simulink model "sldemo_mdlref_variants_enum"  (Simulink 7.6)
settings: Solver=FixedStepDiscrete  StartTime=0.0  StopTime=10.0  RelTol=1e-3
PreLoadFcn:
  | VE_NONLINEAR_CONTROLLER=Simulink.Variant('E_CTRL==sldemo_mrv_CONTROLLER_TYPE.NONLINEAR')
  | VE_SECOND_ORDER_CONTROLLER=Simulink.Variant('E_CTRL==sldemo_mrv_CONTROLLER_TYPE.SECOND_ORDER')
  | 
  | E_CTRL=sldemo_mrv_CONTROLLER_TYPE.SECOND_ORDER
  | 
  | VE_PROTOTYPE = Simulink.Variant('E_CURRENT_BUILD==sldemo_mrv_BUILD_TYPE.PROTOTYPE')
  | VE_PRODUCTION = Simulink.Variant('E_CURRENT_BUILD==sldemo_mrv_BUILD_TYPE.PRODUCTION')
  | 
  | E_CURRENT_BUILD=sldemo_mrv_BUILD_TYPE.PRODUCTION
settings Model: Creator=The MathWorks Inc.
settings DataIOCC: SaveFormat=StructureWithTime
settings OptimizationCC: InlineParams=on
settings RTWCC: ProcessScript=grt_make_rtw_hook
settings CodeAppCC: MaxIdLength=100

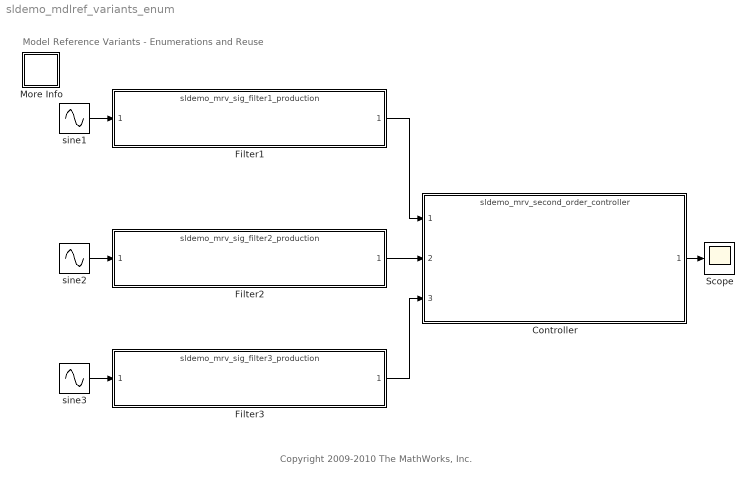
== system sldemo_mdlref_variants_enum ==
  note: Copyright 2009-2010 The MathWorks, Inc.
  note: Model Reference Variants - Enumerations and Reuse
  Controller : ModelReference  ModelNameDialog=sldemo_mrv_second_order_controller  SimulationMode=Normal  Variant=on  ModelReferenceVersion=1.9  CopyOfModelName=sldemo_mrv_second_order_controller
      settings: AttributesFormatString=%<ActiveVariant>
  Filter1 : ModelReference  ModelNameDialog=sldemo_mrv_sig_filter1_production  SimulationMode=Normal  Variant=on  ModelReferenceVersion=1.19  CopyOfModelName=sldemo_mrv_sig_filter1_production
      settings: AttributesFormatString=%<ActiveVariant>
  Filter2 : ModelReference  ModelNameDialog=sldemo_mrv_sig_filter2_production  SimulationMode=Normal  Variant=on  ModelReferenceVersion=1.19  CopyOfModelName=sldemo_mrv_sig_filter2_production
      settings: AttributesFormatString=%<ActiveVariant>
  Filter3 : ModelReference  ModelNameDialog=sldemo_mrv_sig_filter3_production  SimulationMode=Normal  Variant=on  ModelReferenceVersion=1.15  CopyOfModelName=sldemo_mrv_sig_filter3_production
      settings: AttributesFormatString=%<ActiveVariant>
  More Info : Subsystem
      settings: OpenFcn=showdemo('sldemo_mdlref_variants')
      mask Display: disp('?')
  Scope : Scope
  sine1 : Sin  Amplitude=.1  Frequency=pi/3  SampleTime=.01
  sine2 : Sin  Amplitude=2  SampleTime=.01
  sine3 : Sin  Amplitude=.3  Frequency=pi/6  SampleTime=.01
  wires:
  sine2/1 -> Filter2/1
  sine1/1 -> Filter1/1
  sine3/1 -> Filter3/1
  Controller/1 -> Scope/1
  Filter3/1 -> Controller/3
  Filter2/1 -> Controller/2
  Filter1/1 -> Controller/1

== system sldemo_mdlref_variants_enum/More Info ==
  note: Model Reference Variants - Enumerations and Reuse
  note: The following demo illustrates some Simulink.Variant capabilities
      |
      |    1. Enumerations: MATLAB enumeration classes can be used to improve
      |       readability in the conditions of the variant object.
      |
      |    2. Reuse: Simulink.Variant's can be reused in different Model blocks.
